simulink model "sfunction"  (R2024a)
settings: Solver=VariableStepAuto  StartTime=0.0  StopTime=400  RelTol=1e-3
libraries: simulink x2
settings Model: Creator=ericliu  LastModifiedBy=Eason

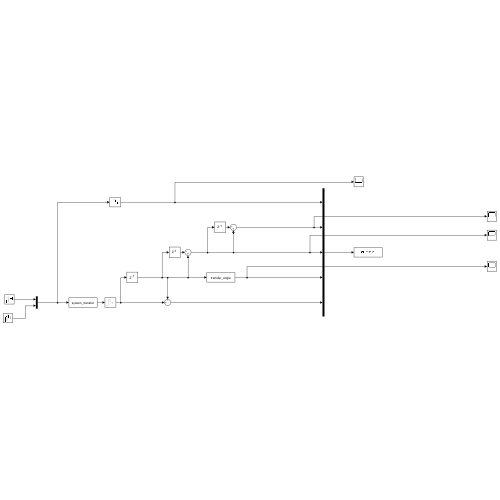
[thumbnail: Simulink's stored preview of the top-level diagram]
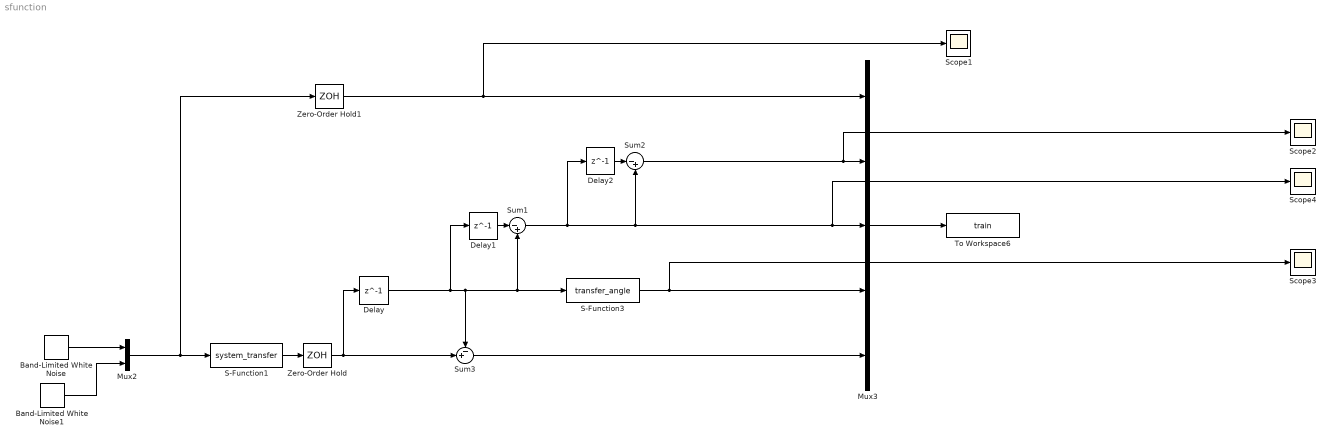
== system sfunction ==
  Band-Limited White Noise : simulink/Sources/Band-Limited White Noise  Cov=[0.004]  Ts=0.001  seed=[23341]
  Band-Limited White Noise1 : simulink/Sources/Band-Limited White Noise  Cov=[0.004]  Ts=0.001  seed=[14695]
  Delay : Delay  DelayLength=1  InitialCondition=0  SampleTime=0.001
  Delay1 : Delay  DelayLength=1  InitialCondition=0  SampleTime=0.001
  Delay2 : Delay  DelayLength=1  InitialCondition=0  SampleTime=0.001
  Mux2 : Mux  Inputs=2
  Mux3 : Mux  Inputs=5
  S-Function1 : S-Function  FunctionName=system_transfer  SFunctionDeploymentMode=off  EnableBusSupport=off
  S-Function3 : S-Function  FunctionName=transfer_angle  SFunctionDeploymentMode=off  EnableBusSupport=off
  Scope{1..4} (4 alike) : Scope
  Sum1 : Sum  Inputs=|-+
  Sum2 : Sum  Inputs=|-+
  Sum3 : Sum  Inputs=-+|
  To Workspace6 : ToWorkspace  VariableName=train  SampleTime=0.01
      settings: Save2DSignal=2-D array (concatenate along first dimension)
  Zero-Order Hold : ZeroOrderHold  SampleTime=0.001
  Zero-Order Hold1 : ZeroOrderHold  SampleTime=0.001
  wires:
  S-Function1/1 -> Zero-Order Hold/1
  Mux2/1 -> Zero-Order Hold1/1, S-Function1/1
  Zero-Order Hold1/1 -> Scope1/1, Mux3/1
  Mux3/1 -> To Workspace6/1
  Band-Limited White Noise/1 -> Mux2/1
  Band-Limited White Noise1/1 -> Mux2/2
  Delay1/1 -> Sum1/1
  Delay2/1 -> Sum2/1
  Delay/1 -> Delay1/1, Sum3/1, S-Function3/1, Sum1/2
  S-Function3/1 -> Scope3/1, Mux3/4
  Sum1/1 -> Delay2/1, Scope4/1, Mux3/3, Sum2/2
  Sum2/1 -> Scope2/1, Mux3/2
  Zero-Order Hold/1 -> Sum3/2, Delay/1
  Sum3/1 -> Mux3/5
